simulink model "PCA1"  (R2018b)
settings: Solver=VariableStepAuto  StartTime=0.0  StopTime=10  RelTol=1e-3
settings Model: Creator=ohara  LastModifiedBy=ohara

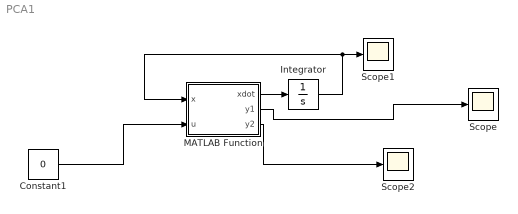
== system PCA1 ==
  Constant1 : Constant  Value=0
  Integrator : Integrator  InitialCondition=[3,3,3,0]
  MATLAB Function : MATLAB Function  TreatAsAtomicUnit=on
  Scope : Scope
  Scope1 : Scope
  Scope2 : Scope
  wires:
  Integrator/1 -> MATLAB Function/1(x), Scope1/1
  MATLAB Function/1(xdot) -> Integrator/1
  MATLAB Function/2(y1) -> Scope/1
  Constant1/1 -> MATLAB Function/2(u)
  MATLAB Function/3(y2) -> Scope2/1

== matlab function PCA1/MATLAB Function ==
  data: x input; xdot output; u input; y1 output; y2 output
function [xdot, y1, y2] = PCA(x, u)
a = 4;
b = 1;
M = 1;
m = 0.4;
g = 9.81;
L = 0.25*M;
xdot1 = x(3);
xdot2 = x(4);
xdot3 = -a*x(3) - ((m*g)/M)*x(2) + b*u;
xdot4 = (a/L)*x(3) - (M+m)*(g/(M*L))*x(2) - (b/L)*u;
xdot  = [xdot1; xdot2; xdot3; xdot4];
y1 = x(1);
y2 = x(2);
